simulink model "q8_sem_deadzone"  (R2025b)
settings: Solver=VariableStepAuto  StartTime=0.0  StopTime=20  RelTol=1e-3
values from neighbouring files (symbols this model uses):
  D_estim = zeros(1,2)    [integrador.m]    (also in q8.m)
  estim_A = A - B*K - L*C    [integrador.m]    (also in q8.m)
  K = lqr(A, B, Qr, Rr)    [IP_MACRO.m]    (also in Integrador_of_IP_MACRO.m = K_aug(1:5); integrador.m = K_aug(1:5))
  L = lqe(A, G, C, Qe, Re)    [IP_MACRO.m]    (also in Integrador_of_IP_MACRO.m; integrador.m; q7.m; q8.m)
  x0 = [0.1 0 0 0 0]'    [integrador.m]    (also in q8.m)
undefined symbols (not defined in the file or in its folder): A, B, C, D
settings Model: Creator=matos  LastModifiedBy=matos

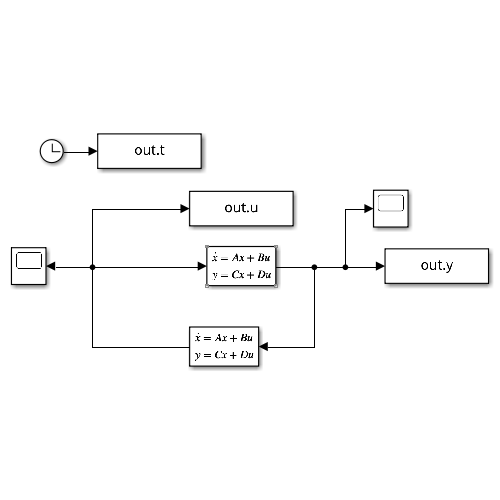
[thumbnail: Simulink's stored preview of the top-level diagram]
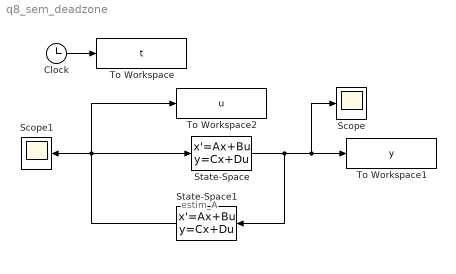
== system q8_sem_deadzone ==
  note: estim_A
  Clock : Clock
  Scope : Scope
      settings: ActiveDisplayYMinimum=-0.018324001872298344  ActiveDisplayYMaximum=0.12112647393831649
  Scope1 : Scope
  State-Space : StateSpace  A=A  B=B  C=C  D=D  InitialCondition=x0
  State-Space1 : StateSpace  A=estim_A  B=L  C=-K  D=D_estim  InitialCondition=0
  To Workspace : ToWorkspace  VariableName=t  SaveFormat=Timeseries  SampleTime=-1
  To Workspace1 : ToWorkspace  VariableName=y  SaveFormat=Timeseries  SampleTime=-1
  To Workspace2 : ToWorkspace  VariableName=u  SaveFormat=Timeseries  SampleTime=-1
  wires:
  Clock/1 -> To Workspace/1
  State-Space/1 -> Scope/1, To Workspace1/1, State-Space1/1
  State-Space1/1 -> To Workspace2/1, Scope1/1, State-Space/1
